simulink model "linearLatDir"  (R2021b)
settings: Solver=VariableStepAuto  StartTime=0.0  StopTime=5  RelTol=1e-3
libraries: slpidlib x1
settings Model: Creator=pablo  LastModifiedBy=jakub
settings SolverCC: AlgebraicLoopSolver=TrustRegion
settings DebuggingCC: SFMachineParentedDataDiag=warning  ArithmeticOperatorsInVariantConditions=warning
settings SFSimCC: CustomCodeUndefinedFunction=UseInterfaceOnly

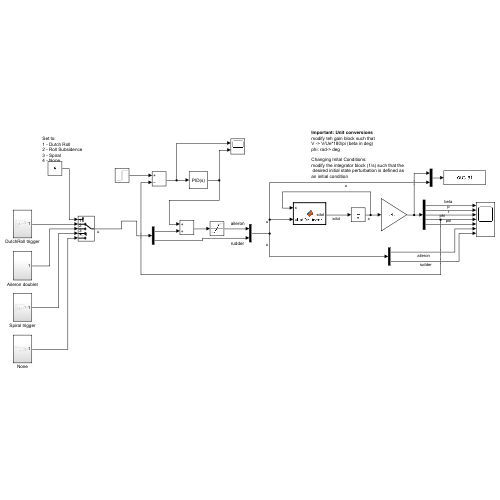
[thumbnail: Simulink's stored preview of the top-level diagram]
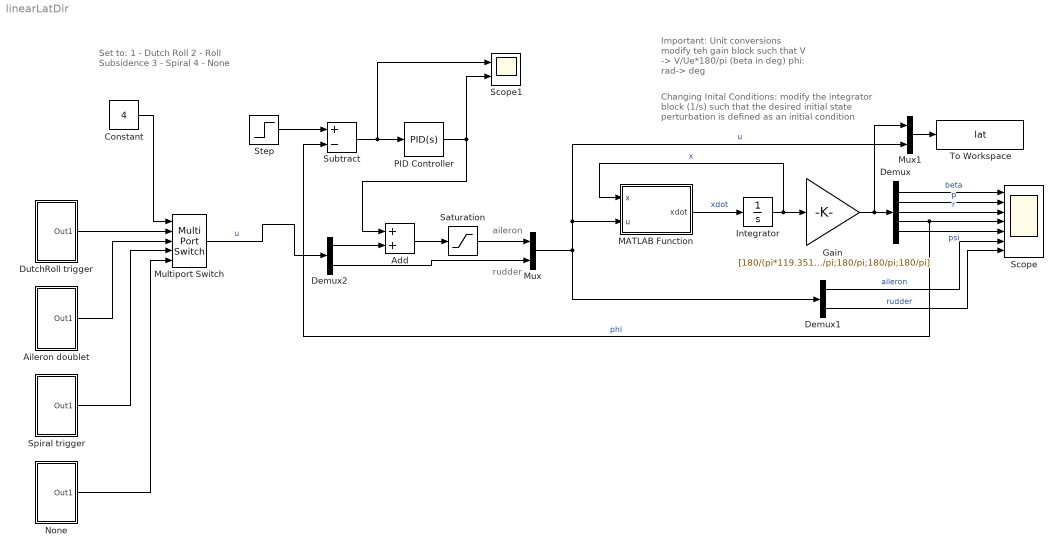
== system linearLatDir ==
  note: rudder
  note: aileron
  note: Set to:
      | 1 - Dutch Roll
      | 2 - Roll Subsidence
      | 3 - Spiral
      | 4 - None
  note: Important: Unit conversions
      | modify teh gain block such that
      | V -> V/Ue*180/pi (beta in deg)
      | phi: rad-> deg
  note: Changing Inital Conditions:
      | modify the integrator block (1/s) such that the
      | desired initial state perturbation is defined as
      | an initial condition
  Add : Sum
  Aileron doublet : Subsystem
  Constant : Constant  Value=4
  Demux : Demux  Outputs=5
  Demux1 : Demux  Outputs=2
  Demux2 : Demux  Outputs=2
  DutchRoll trigger : Subsystem
  Gain : Gain  Gain=[180/(pi*119.351);180/pi;180/pi;180/pi;180/pi]
  Integrator : Integrator  InitialCondition=[0;0;0;-15*pi/180;0]
  MATLAB Function : MATLAB Function  TreatAsAtomicUnit=on
  Multiport Switch : MultiPortSwitch  Inputs=4
  Mux : Mux  Inputs=2
  Mux1 : Mux  Inputs=2
  None : Subsystem
  PID Controller : slpidlib/PID Controller  Controller=PID  Form=Parallel  TimeDomain=Continuous-time  UseExternalTs=off  SampleTime=-1  IntegratorMethod=Forward Euler  FilterMethod=Forward Euler  ControllerParametersSource=internal  P=-0.07  I=0  D=0  UseFilter=on  N=100  TunerSelectOption=Transfer Function Based (PID Tuner App)  InitialConditionSource=internal  InitialConditionForIntegrator=0  InitialConditionForFilter=0  DifferentiatorICPrevScaledInput=0  ExternalReset=none  TrackingMode=off  Kt=1  LimitOutput=off  SatLimitsSource=internal  UpperSaturationLimit=inf  LowerSaturationLimit=-inf  LinearizeAsGain=on  AntiWindupMode=none  Kb=1  POutMin=[]  POutMax=[]  IOutMin=[]  IOutMax=[]  DOutMin=[]  DOutMax=[]  NOutMin=[]  NOutMax=[]  SumOutMin=[]  SumOutMax=[]  SaturationOutMin=[]  SaturationOutMax=[]  PParamMin=[]  PParamMax=[]  IParamMin=[]  IParamMax=[]  DParamMin=[]  DParamMax=[]  NParamMin=[]  NParamMax=[]  KbParamMin=[]  KbParamMax=[]  KtParamMin=[]  KtParamMax=[]  KbOutMin=[]  KbOutMax=[]  KtOutMin=[]  KtOutMax=[]  IntegratorOutMin=[]  IntegratorOutMax=[]  FilterOutMin=[]  FilterOutMax=[]  SumI1OutMin=[]  SumI1OutMax=[]  SumI2OutMin=[]  SumI2OutMax=[]  SumI3OutMin=[]  SumI3OutMax=[]  SumI4OutMin=[]  SumI4OutMax=[]  SumDOutMin=[]  SumDOutMax=[]  DifferentiatorOutMin=[]  DifferentiatorOutMax=[]  FilterDiffOutCoefMin=[]  FilterDiffOutCoefMax=[]  ReciprocalOutMin=[]  ReciprocalOutMax=[]  SumDenOutMin=[]  SumDenOutMax=[]  SumNumOutMin=[]  SumNumOutMax=[]  DivideOutMin=[]  DivideOutMax=[]  UdiffTsProdOutMin=[]  UdiffTsProdOutMax=[]  NTsProdOutMin=[]  NTsProdOutMax=[]  UintegralTsProdOutMin=[]  UintegralTsProdOutMax=[]  UngainTsProdOutMin=[]  UngainTsProdOutMax=[]  IntegratorContinuousStateAttributes=''  IntegratorStateMustResolveToSignalObject=off  IntegratorRTWStateStorageClass=Auto  FilterContinuousStateAttributes=''  FilterStateMustResolveToSignalObject=off  FilterRTWStateStorageClass=Auto  ParallelPVariant=InternalParameters  IdealPVariant=Disabled  IVariant=InternalParameters  DVariant=InternalParameters  IntegratorVariant=Continuous  SatVariant=Disabled  AWVariant=Passthrough  PCopyVariant=Disabled  TRVariant=Disabled  FdbkBlocksVariant=Forward  IdealPFdbkVariant=Disabled  SatFdbkVariant=Disabled  DerivativeFilterVariant=ContFilter  NVariant=InternalParameters  NCopyVariant=Disabled  FilterICVariant=InternalICsFilter  IntegratorICVariant=InternalICs  ExternalResetVariant=Disabled  TRSumVariant=Passthrough  SumFdbkVariant=Disabled  SumVariant=Sum_PID  TsampFilterVariant=InternalTs  TsampNgainVariant=Passthrough  TsampIntegralVariant=Passthrough  ExternalSaturationOutDataTypeStr=Inherit: Same as second input
  Saturation : Saturate  UpperLimit=1  LowerLimit=-1
  Scope : Scope  NumInputPorts=7
  Scope1 : Scope  NumInputPorts=2
  Spiral trigger : Subsystem
  Step : Step  After=0  SampleTime=0
  Subtract : Sum  Inputs=+-
  To Workspace : ToWorkspace  VariableName=lat  SaveFormat=Timeseries  SampleTime=0.01
  wires:
  MATLAB Function/1(xdot) -> Integrator/1  "xdot"
  Integrator/1 -> MATLAB Function/1(x), Gain/1  "x"
  Gain/1 -> Mux1/1, Demux/1
  Demux/1 -> Scope/1  "beta"
  Demux/2 -> Scope/2  "p"
  Demux/3 -> Scope/3  "r"
  Demux/4 -> Scope/4, Subtract/2  "phi"
  DutchRoll trigger/1(Out1) -> Multiport Switch/2
  Demux1/1 -> Scope/6  "aileron"
  Demux1/2 -> Scope/7  "rudder"
  Mux1/1 -> To Workspace/1
  Mux/1 -> Demux1/1, MATLAB Function/2(u), Mux1/2  "u"
  Aileron doublet/1(Out1) -> Multiport Switch/3
  Spiral trigger/1(Out1) -> Multiport Switch/4
  Constant/1 -> Multiport Switch/1
  Demux/5 -> Scope/5  "psi"
  None/1(Out1) -> Multiport Switch/5
  Demux2/2 -> Mux/2
  PID Controller/1 -> Scope1/2, Add/1
  Subtract/1 -> Scope1/1, PID Controller/1
  Step/1 -> Subtract/1
  Multiport Switch/1 -> Demux2/1  "u"
  Demux2/1 -> Add/2
  Add/1 -> Saturation/1
  Saturation/1 -> Mux/1

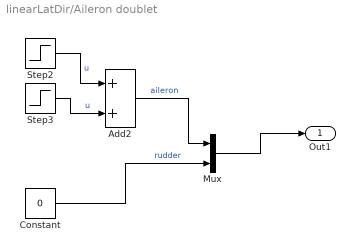
== system linearLatDir/Aileron doublet ==
  Add2 : Sum
  Constant : Constant  Value=0
  Mux : Mux  Inputs=2
  Step2 : Step  Time=0.8  SampleTime=0
  Step3 : Step  Time=1.6  After=-1  SampleTime=0
  Out1 : Outport  VectorParamsAs1DForOutWhenUnconnected=off
  wires:
  Mux/1 -> Out1/1
  Add2/1 -> Mux/1  "aileron"
  Step2/1 -> Add2/1  "u"
  Constant/1 -> Mux/2  "rudder"
  Step3/1 -> Add2/2  "u"

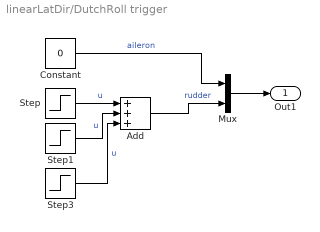
== system linearLatDir/DutchRoll trigger ==
  Add : Sum  Inputs=+++
  Constant : Constant  Value=0
  Mux : Mux  Inputs=2
  Step : Step  Time=0.6  SampleTime=0
  Step1 : Step  Time=1.2  After=-2  SampleTime=0
  Step3 : Step  Time=1.8  SampleTime=0
  Out1 : Outport
  wires:
  Add/1 -> Mux/2  "rudder"
  Step1/1 -> Add/2  "u"
  Step/1 -> Add/1  "u"
  Constant/1 -> Mux/1  "aileron"
  Mux/1 -> Out1/1
  Step3/1 -> Add/3  "u"

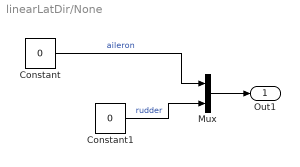
== system linearLatDir/None ==
  Constant : Constant  Value=0
  Constant1 : Constant  Value=0
  Mux : Mux  Inputs=2
  Out1 : Outport
  wires:
  Constant1/1 -> Mux/2  "rudder"
  Constant/1 -> Mux/1  "aileron"
  Mux/1 -> Out1/1

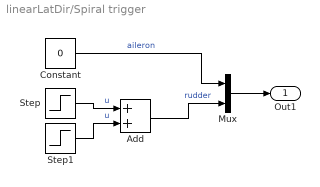
== system linearLatDir/Spiral trigger ==
  Add : Sum
  Constant : Constant  Value=0
  Mux : Mux  Inputs=2
  Step : Step  Time=0.6  SampleTime=0
  Step1 : Step  Time=1.2  After=-1  SampleTime=0
  Out1 : Outport
  wires:
  Add/1 -> Mux/2  "rudder"
  Step1/1 -> Add/2  "u"
  Step/1 -> Add/1  "u"
  Constant/1 -> Mux/1  "aileron"
  Mux/1 -> Out1/1

== matlab function linearLatDir/MATLAB Function ==
  data: x input; u input; xdot output
function xdot = LatDirLinear(x,u)
%inputs - x: (5x1)lateral state vector
%         x(1)- v   m/s
%         x(2)- p   rad/s
%         x(3)- r   rad/s
%         x(4)- phi rad
%         x(5)- psi rad
%       - u: lateral control vector
%         u(1)- aileron deflection as percentage
%         u(2)- rudder deflection as percentage
%Outputs-xdot:(5x1)
%Define parameters for aircraft
m = 9.2700e+03; %kg
Ixx = 4.5547e+04;%kg m^2
Izx = 119.9222;%kg m^2
Izz = 1.4903e+05;%kg m^2
Ue = 114.7211;%m/s
g = 9.81; %m/s^2
theta = 0; %rad

Yv = -2.2192e+03; %Ns/m
Yp = 1.3693e+03; %Ns
Yr = 1.0568e+04; %Ns
Lv = -5.8237e+03; %Ns
Lp = -3.7598e+05; %Nms
Lr = 1.3196e+05; %Nms
Nv = 6.2265e+03; %Ns
Np = -2.0419e+04; %Nms
Nr = -1.0884e+05; %Nms
%Aileron input
Y_a = 0; 
L_a = -7.0507e+05; %Rolling moment due to aileron deflection in RAD - Nm
N_a = 0;
%Rudder input
Y_r = 1.3630e+05; %Sideforce derivative with rudder in RAD - Nm
L_r = 1.3630e+05; %Rolling moment derivative with rudder in RAD - Nm
N_r = -1.0322e+06; %Yawing moment derivative with rudder in RAD - Nm

M = [   m,  0,  0,  0,  0;
        0,  Ixx,-Izx,0, 0;
        0,  -Izx,Izz,0, 0;
        0,  0,  0,  1,  0;
        0,  0,  0,  0,  1];

A = [   Yv,     Yp,     Yr-m*Ue,    m*g*cos(theta), 0;
        Lv,     Lp,     Lr,         0,              0;
        Nv,     Np,     Nr,         0,              0;
        0,      1,      tan(theta), 0,              0;
        0,      0,      sec(theta), 0,              0];

B = [   Y_a,    Y_r;
        L_a,    L_r;
        N_a,    N_r;
        0,      0;
        0,      0];

u=u.*[25;-30]*pi/180; %convert percentage to angle in rad
xdot = M\(A*x+B*u);
